simulink model "pend"  (R2021a)
settings: Solver=ode45  StartTime=0.0  StopTime=Tfinal  RelTol=1e-3  EnableMultiTasking=on
values from neighbouring files (symbols this model uses):
  Ts = 0.1    [Copy_of_salida.mat]    (also in P3.m)
  x0 = x_next    [P3.m]    (also in P3_old.m = [0; 0; pi+0.01;0]; control_cart.m = x_control(:,k+1))
settings Model: Creator=Pendulo  LastModifiedBy=sebag
settings SolverCC: AlgebraicLoopSolver=TrustRegion
settings DataIOCC: LimitDataPoints=on  SaveFormat=Array  ReturnWorkspaceOutputs=off
settings OptimizationCC: LifeSpan=inf
settings DebuggingCC: UnderspecifiedInitializationDetection=Classic  MergeDetectMultiDrivingBlocksExec=none  SolverPrmCheckMsg=warning  SFUnexpectedBacktrackingDiag=warning  SFNoUnconditionalDefaultTransitionDiag=warning  SFExecutionAtInitializationDiag=none  SFMachineParentedDataDiag=warning  ArithmeticOperatorsInVariantConditions=warning
settings HardwareCC: ProdBitPerPointer=32  ProdBitPerSizeT=32  ProdBitPerPtrDiffT=32  ProdLargestAtomicFloat=None  ProdIntDivRoundTo=Undefined  ProdEndianess=Unspecified  ProdWordSize=32  ProdHWDeviceType=32-bit Generic
settings ModelReferenceCC: PropagateSignalLabelsOutOfModel=off
settings SFSimCC: SimUseLocalCustomCode=off  CustomCodeUndefinedFunction=UseInterfaceOnly
settings RTWCC: RTWUseLocalCustomCode=off
settings CodeAppCC: StateflowObjectComments=on
settings GRTTargetCC: TargetLangStandard=C89/C90 (ANSI)
settings ConfigComp: CovMetricSettings=dw  CovSaveCumulativeToWorkspaceVar=on  CovSaveSingleToWorkspaceVar=on  CovExternalEMLEnable=off

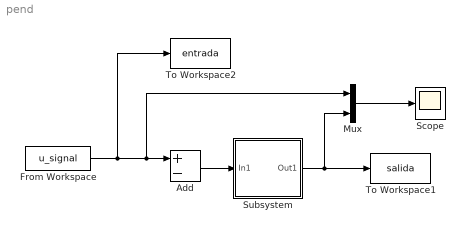
== system pend ==
  Add : Sum  Inputs=+-
  From Workspace : FromWorkspace  VariableName=u_signal  SampleTime=Ts
  Mux : Mux  Inputs=2
  Scope : Scope
  Subsystem : Subsystem
  To Workspace1 : ToWorkspace  VariableName=salida  SampleTime=Ts
  To Workspace2 : ToWorkspace  VariableName=entrada  SampleTime=Ts
  wires:
  Subsystem/1(Out1) -> To Workspace1/1, Mux/2
  From Workspace/1 -> To Workspace2/1, Mux/1, Add/1
  Mux/1 -> Scope/1
  Add/1 -> Subsystem/1(In1)

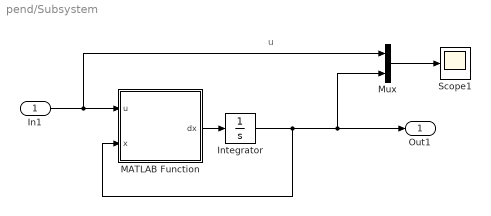
== system pend/Subsystem ==
  note: u
  In1 : Inport
  Integrator : Integrator  InitialCondition=x0
  MATLAB Function : MATLAB Function  TreatAsAtomicUnit=on
  Mux : Mux  Inputs=2
  Scope1 : Scope
  Out1 : Outport
  wires:
  MATLAB Function/1(dx) -> Integrator/1
  In1/1 -> Mux/1, MATLAB Function/1(u)
  Integrator/1 -> MATLAB Function/2(x), Out1/1, Mux/2
  Mux/1 -> Scope1/1

== matlab function pend/Subsystem/MATLAB Function ==
  data: u input; x input; dx output
function dx = pendcart(u,x)
%x=[x,dx,theta,dtheta]


m = 1;
M = 5;
L = 2;
g = -9.8;
d = 1;



Sx = sin(x(3));
Cx = cos(x(3));
D = L*(M+m*(1-Cx^2));

dx=[x(2);(1/D)*(-m*L*g*Cx*Sx + L*(m*L*x(4)^2*Sx - d*x(2)) + L*u);...
    x(4);(1/D)*((m+M)*g*Sx - Cx*(m*L*x(4)^2*Sx - d*x(2)) - Cx*u)];
